simulink model "DC_Series_Wound_New_Simulation"  (R2021a)
settings: Solver=VariableStepAuto  StartTime=0.0  StopTime=10.0  RelTol=1e-3
values from neighbouring files (symbols this model uses):
  A = 0.1    [Kibble_Simu_4.m]    (also in Kibble_Simulation_code2.m; LQG.m = [1.1269   -0.4940    0.1129; LQG_TEST2.m = [0 1 0 0; LQR.m = [0 1 0 0)
  N = 0    [LQG.m]    (also in LQG_TEST2.m; LQR.m = [0; 0; 0;0])
libraries: spsDCMachineLib x1, spsDCVoltageSourceLib x1, spspowerguiLib x1
settings Model: Creator=HP  LastModifiedBy=HP

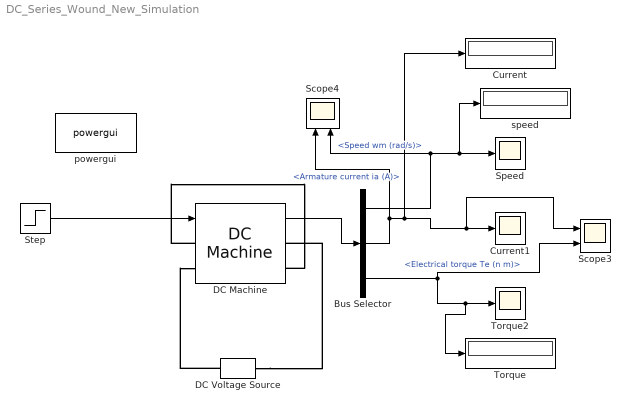
== system DC_Series_Wound_New_Simulation ==
  Bus Selector : BusSelector  OutputSignals=Speed wm (rad/s),Armature current ia (A),Electrical torque Te (n m)
  Current : Display
  Current1 : Scope
  DC Machine : spsDCMachineLib/DC Machine  PresetModel=01: 5HP 240V 1750RPM Field:300V  MechanicalLoad=Torque TL  FieldType=Wound  ShowDetailedParameters=on  MeasurementBus=off  RLa=[2.581 0.028]  RLf=[281.2 156]  Laf=0.9483  MachineConstant=Torque constant (N.m/A)  Ke=1.8  Kt=1.8  J=0.02215  Bm=0.002953  Tf=0.5161  w0=1  Ifinit=1.05715322731261  TsPowergui=0  TsBlock=-1
  DC Voltage Source : spsDCVoltageSourceLib/DC Voltage Source  Amplitude=300  Measurements=None
  Scope3 : Scope  NumInputPorts=2
  Scope4 : Scope  NumInputPorts=2
  Speed : Scope
  Step : Step  Time=20  SampleTime=0
  Torque : Display
  Torque2 : Scope
  powergui : spspowerguiLib/powergui  Priority=1  SimulationMode=Continuous  SampleTime=50e-6  frequency=60  Iterations=50  frequencyindice=0  Pbase=100e6  ErrMax=1e-4  UnitsV=kV  UnitsW=MW  buscounter=0  FunctionMessages=off  echomessages=off  EnableUseOfTLC=off  CurrentSourceSwitches=off  DisableSnubberDevices=off  DisableRonSwitches=off  DisableVfSwitches=off  DisplayEquations=off  AutomaticDiscreteSolvers=off  SolverType=Tustin/Backward Euler (TBE)  Interpol=off  ExternalGateDelay=off  methode=off  Ts=100  x0status=blocks  SPID=on  SwTol=0  HookPort=off  NonlinearTolerance=1e-4  nMaxIteration=100  ContinueOnMaxIteration=off  RestoreLinks=warning  ResistiveCurrentMeasurement=off  Frange=[0:2:500]  Ylog=off  Xlog=on  ShowGrid=off  save=off  variable=ZData  structure=0  ZoomFFT=off  StartTime=0.0  cycles=1  DisplayStyle=1  fundamental=60  FreqAxis=off  MaxFrequency=1000  frequencyindicesteady=1  RmsSteady=1  display=off
  speed : Display
  wires:
  DC Machine/1 -> Bus Selector/1
  Bus Selector/1 -> Scope4/2, speed/1, Speed/1  "<Speed wm (rad/s)>"
  Bus Selector/2 -> Current/1, Scope3/1, Current1/1, Scope4/1  "<Armature current ia (A)>"
  Bus Selector/3 -> Scope3/2, Torque/1, Torque2/1  "<Electrical torque Te (n m)>"
  Step/1 -> DC Machine/1
  connections:
  DC Voltage Source/RConn1 -- DC Machine/LConn2
  DC Voltage Source/LConn1 -- DC Machine/RConn1
  DC Machine/LConn1 -- DC Machine/RConn2
